simulink model "sim_robot_control"  (R2019b)
settings: Solver=VariableStepAuto  StartTime=0.0  StopTime=T_tot  FixedStep=0.0001  RelTol=1e-3
model workspace: external: MATLAB File G:\Drive condivisi\SSR_project\cad\modello_ultimo\sim\robot_DataFile.m (data not in the file)
values from neighbouring files (symbols this model uses):
  m = m + 1    (= 2)    [computa_singolarita.m]    (also in computa_ws3D.m; plot_ws_2D_viste.m = 14)
  X = []    [computa_singolarita.m]    (also in computa_ws3D.m; pianificazione_traiettoria.m = Q+[r*sqrt(2),0,-r*sqrt(2)]; pianificazione_traiettoria_grafici.m = Q+[r*sqrt(2),0,-r*sqrt(2)]; plotCylinderWithCaps.m = X + cnt(1))
  Y = []    [computa_singolarita.m]    (also in computa_ws3D.m; pianificazione_traiettoria.m = X+[r-0.05*r,0,r-0.05*r]; pianificazione_traiettoria_grafici.m = X+[r-0.05*r,0,r-0.05*r]; plotCylinderWithCaps.m = Y + cnt(2))
  Z = []    [computa_singolarita.m]    (also in computa_ws3D.m; plotCylinderWithCaps.m = Z * height; plot_ws_2D_viste.m)
undefined symbols (not defined in the file or in its folder): sigbuilder_block, smiData
libraries: sm_lib x40, nesl_utility x28
(part 2 of 2)

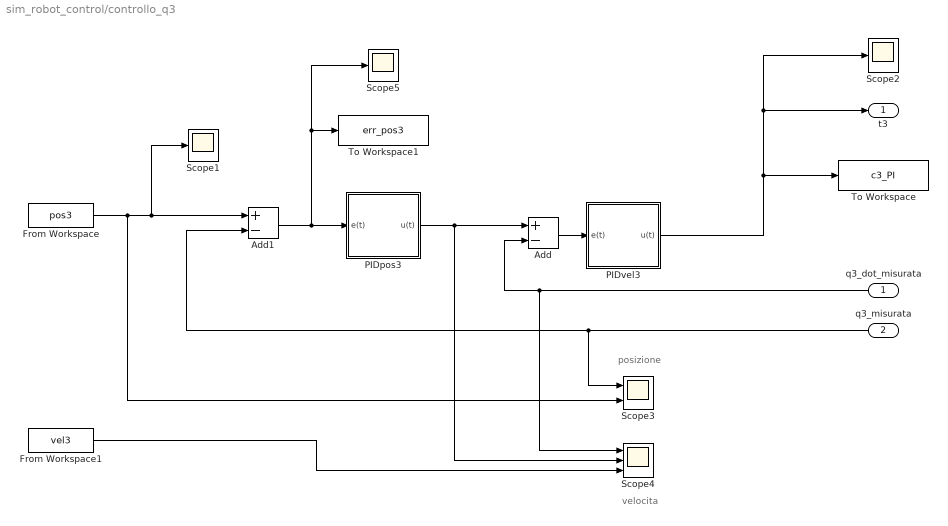
== system sim_robot_control/controllo_q3 ==
  note: velocita
  note: posizione
  q3_dot_misurata : Inport
  q3_misurata : Inport  Port=2
  Add : Sum  Inputs=+-
  Add1 : Sum  Inputs=+-
  From Workspace : FromWorkspace  VariableName=pos3  SampleTime=0
  From Workspace1 : FromWorkspace  VariableName=vel3  SampleTime=0
  "PIDpos3 " : Subsystem  mask(PID){Kp=30, Ti=8, Td=0, sp_w=0.6}
      mask help: Standard formulation
  PIDvel3 : Subsystem  mask(PID){Kp=100, Ti=10, Td=0, sp_w=0.7}
      mask help: Standard formulation
  Scope1 : Scope
  Scope2 : Scope
  Scope3 : Scope  NumInputPorts=2
  Scope4 : Scope  NumInputPorts=3
  Scope5 : Scope
  To Workspace : ToWorkspace  VariableName=c3_PI  SampleTime=-1
      settings: Save2DSignal=2-D array (concatenate along first dimension)
  To Workspace1 : ToWorkspace  VariableName=err_pos3  SampleTime=-1
      settings: Save2DSignal=2-D array (concatenate along first dimension)
  t3 : Outport
  wires:
  q3_misurata/1 -> Scope3/1, Add1/2
  Add/1 -> PIDvel3/1(e(t))
  q3_dot_misurata/1 -> Scope4/1, Add/2
  Add1/1 -> Scope5/1, To Workspace1/1, "PIDpos3 "/1(e(t))
  From Workspace/1 -> Scope3/2, Scope1/1, Add1/1
  PIDvel3/1(u(t)) -> To Workspace/1, Scope2/1, t3/1
  From Workspace1/1 -> Scope4/3
  "PIDpos3 "/1(u(t)) -> Scope4/2, Add/1

== system sim_robot_control/massa pezzo ==
  Demux : Demux  Tag=STV Demux  Outputs=1
  FromWs : FromWorkspace  Tag=STV FromWs  VariableName=tuvar  SampleTime=0
      SigBuilderData=|
      | common.afterFinalStr = 'Extrapolate'
      | common.sampleTime = 0
      | dataSet.timeRange = [0 57.824]
      | dataSet.name = 'Group 1'
      | sbobj.Groups.Name = 'Group 1'
      | sbobj.Groups.Signals.Name = 'massa pz'
      | sbobj.Groups.Signals.XData = [0 6.412 6.412 51.412 51.412 57.824]
      | sbobj.Groups.Signals.YData = [0 0 1 1 0 0]
      | sbobj.Groups.TimeRange = [0 57.824]
  massa pz : Outport  Tag=STV Outport
  wires:
  FromWs/1 -> Demux/1
  Demux/1 -> massa pz/1

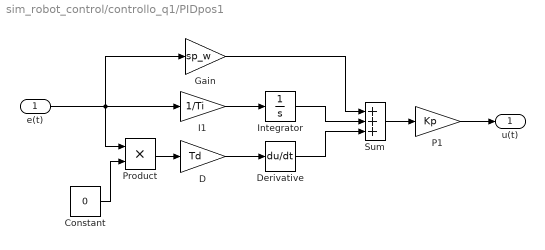
== system sim_robot_control/controllo_q1/PIDpos1 ==
  e(t) : Inport
  Constant : Constant  Value=0
  D : Gain  Gain=Td
  Derivative : Derivative
  Gain : Gain  Gain=sp_w
  I1 : Gain  Gain=1/Ti
  Integrator : Integrator
  P1 : Gain  Gain=Kp
  Product : Product
  Sum : Sum  Inputs=+++
  u(t) : Outport  VectorParamsAs1DForOutWhenUnconnected=off
  wires:
  I1/1 -> Integrator/1
  Integrator/1 -> Sum/2
  D/1 -> Derivative/1
  Derivative/1 -> Sum/3
  e(t)/1 -> Product/1, I1/1, Gain/1
  P1/1 -> u(t)/1
  Sum/1 -> P1/1
  Gain/1 -> Sum/1
  Product/1 -> D/1
  Constant/1 -> Product/2

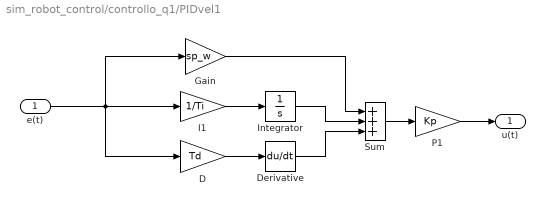
== system sim_robot_control/controllo_q1/PIDvel1 ==
  e(t) : Inport
  D : Gain  Gain=Td
  Derivative : Derivative
  Gain : Gain  Gain=sp_w
  I1 : Gain  Gain=1/Ti
  Integrator : Integrator
  P1 : Gain  Gain=Kp
  Sum : Sum  Inputs=+++
  u(t) : Outport  VectorParamsAs1DForOutWhenUnconnected=off
  wires:
  Gain/1 -> Sum/1
  Sum/1 -> P1/1
  P1/1 -> u(t)/1
  e(t)/1 -> I1/1, Gain/1, D/1
  Derivative/1 -> Sum/3
  D/1 -> Derivative/1
  Integrator/1 -> Sum/2
  I1/1 -> Integrator/1

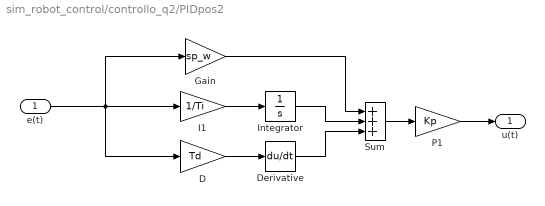
== system sim_robot_control/controllo_q2/PIDpos2  ==
  e(t) : Inport
  D : Gain  Gain=Td
  Derivative : Derivative
  Gain : Gain  Gain=sp_w
  I1 : Gain  Gain=1/Ti
  Integrator : Integrator
  P1 : Gain  Gain=Kp
  Sum : Sum  Inputs=+++
  u(t) : Outport  VectorParamsAs1DForOutWhenUnconnected=off
  wires:
  I1/1 -> Integrator/1
  Integrator/1 -> Sum/2
  D/1 -> Derivative/1
  Derivative/1 -> Sum/3
  e(t)/1 -> I1/1, D/1, Gain/1
  P1/1 -> u(t)/1
  Sum/1 -> P1/1
  Gain/1 -> Sum/1

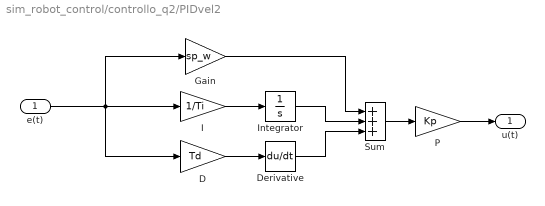
== system sim_robot_control/controllo_q2/PIDvel2 ==
  e(t) : Inport
  D : Gain  Gain=Td
  Derivative : Derivative
  Gain : Gain  Gain=sp_w
  I : Gain  Gain=1/Ti
  Integrator : Integrator
  P : Gain  Gain=Kp
  Sum : Sum  Inputs=+++
  u(t) : Outport  VectorParamsAs1DForOutWhenUnconnected=off
  wires:
  Gain/1 -> Sum/1
  Sum/1 -> P/1
  P/1 -> u(t)/1
  e(t)/1 -> Gain/1, I/1, D/1
  Derivative/1 -> Sum/3
  D/1 -> Derivative/1
  Integrator/1 -> Sum/2
  I/1 -> Integrator/1

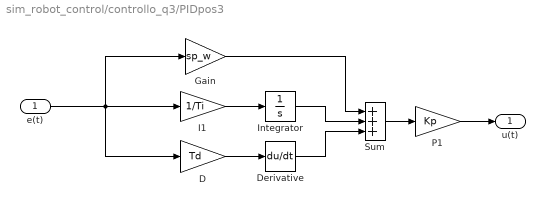
== system sim_robot_control/controllo_q3/PIDpos3  ==
  e(t) : Inport
  D : Gain  Gain=Td
  Derivative : Derivative
  Gain : Gain  Gain=sp_w
  I1 : Gain  Gain=1/Ti
  Integrator : Integrator
  P1 : Gain  Gain=Kp
  Sum : Sum  Inputs=+++
  u(t) : Outport  VectorParamsAs1DForOutWhenUnconnected=off
  wires:
  I1/1 -> Integrator/1
  Integrator/1 -> Sum/2
  D/1 -> Derivative/1
  Derivative/1 -> Sum/3
  e(t)/1 -> I1/1, D/1, Gain/1
  P1/1 -> u(t)/1
  Sum/1 -> P1/1
  Gain/1 -> Sum/1

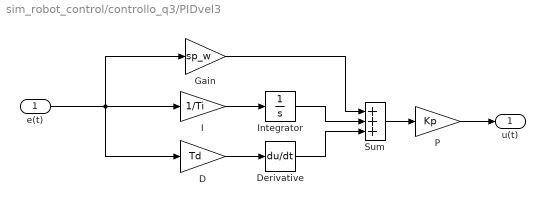
== system sim_robot_control/controllo_q3/PIDvel3 ==
  e(t) : Inport
  D : Gain  Gain=Td
  Derivative : Derivative
  Gain : Gain  Gain=sp_w
  I : Gain  Gain=1/Ti
  Integrator : Integrator
  P : Gain  Gain=Kp
  Sum : Sum  Inputs=+++
  u(t) : Outport  VectorParamsAs1DForOutWhenUnconnected=off
  wires:
  I/1 -> Integrator/1
  Integrator/1 -> Sum/2
  D/1 -> Derivative/1
  Derivative/1 -> Sum/3
  e(t)/1 -> D/1, I/1, Gain/1
  P/1 -> u(t)/1
  Sum/1 -> P/1
  Gain/1 -> Sum/1
